simulink subsystem "HI_SPI"  (R2019b)
settings: Solver=VariableStepAuto  StartTime=0.0  StopTime=10.0  RelTol=1e-3
libraries: hdlsllib x1, c280xlib x1
settings Model: Creator=Nick  LastModifiedBy=Nick

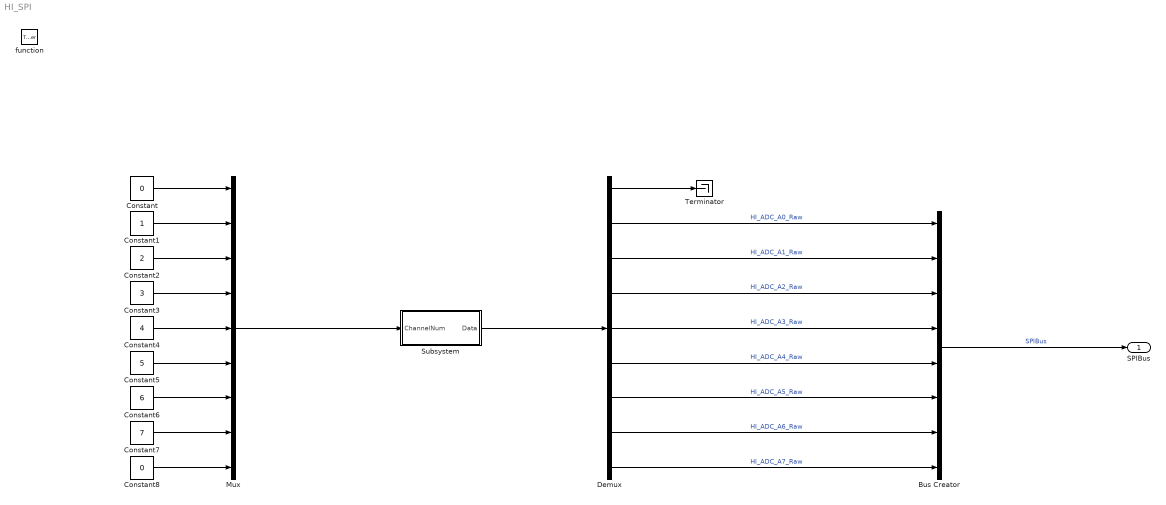
== system HI_SPI ==
  function : TriggerPort  TriggerType=function-call  VariantControl=Variant
  Bus Creator : BusCreator  Inputs=8
  Constant : Constant  Value=0
  Constant1 : Constant
  Constant2 : Constant  Value=2
  Constant3 : Constant  Value=3
  Constant4 : Constant  Value=4
  Constant5 : Constant  Value=5
  Constant6 : Constant  Value=6
  Constant7 : Constant  Value=7
  Constant8 : Constant  Value=0
  Demux : Demux  Outputs=9
  Mux : Mux  Inputs=9
  Subsystem : Subsystem
  Terminator : Terminator
  SPIBus : Outport
  wires:
  Demux/9 -> Bus Creator/8  "HI_ADC_A7_Raw"
  Demux/8 -> Bus Creator/7  "HI_ADC_A6_Raw"
  Demux/7 -> Bus Creator/6  "HI_ADC_A5_Raw"
  Demux/6 -> Bus Creator/5  "HI_ADC_A4_Raw"
  Demux/5 -> Bus Creator/4  "HI_ADC_A3_Raw"
  Demux/4 -> Bus Creator/3  "HI_ADC_A2_Raw"
  Demux/3 -> Bus Creator/2  "HI_ADC_A1_Raw"
  Demux/2 -> Bus Creator/1  "HI_ADC_A0_Raw"
  Demux/1 -> Terminator/1
  Subsystem/1(Data) -> Demux/1
  Mux/1 -> Subsystem/1(ChannelNum)
  Constant8/1 -> Mux/9
  Constant7/1 -> Mux/8
  Constant6/1 -> Mux/7
  Constant5/1 -> Mux/6
  Constant4/1 -> Mux/5
  Constant/1 -> Mux/1
  Constant1/1 -> Mux/2
  Constant2/1 -> Mux/3
  Constant3/1 -> Mux/4
  Bus Creator/1 -> SPIBus/1  "SPIBus"

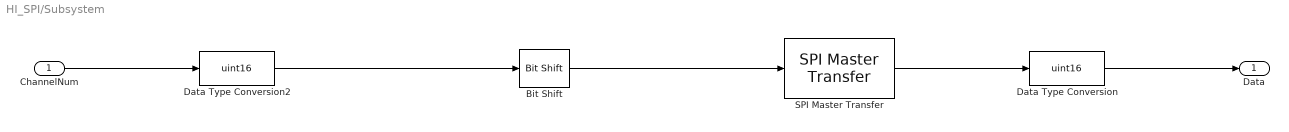
== system HI_SPI/Subsystem ==
  ChannelNum : Inport
  Bit Shift : hdlsllib/Logic and Bit Operations/Bit Shift  mode=Shift Left Logical  N=11
      settings: SourceProductName=Simulink
  Data Type Conversion : DataTypeConversion  OutDataTypeStr=uint16
  Data Type Conversion2 : DataTypeConversion  OutDataTypeStr=uint16
  SPI Master Transfer : c280xlib/SPI Master Transfer  SPISelect=SPI_B  ClockPolarity=Falling_edge  ClockPhase=No_delay  SPIModule=uint32(0)  Mode=Master  BusSpeed=uint32(1000000)  FirstBitToTransfer=Most significant bit (MSB)  ClockMode=0  BlockFunction=Transfer  EnableRegisterAddress=on  RegisterAddress=0  OutputDataType=int8  OutputDataLength=1  DataBits=16  UseCustomSSPin=Explicit GPIO calls  ActiveLowSSPin=Active low  Pin=66
      settings: SourceProductName=Embedded Coder Support Package for Texas Instruments C2000 Processors  SourceProductBaseCode=TIC2000
  Data : Outport
  wires:
  ChannelNum/1 -> Data Type Conversion2/1
  Data Type Conversion/1 -> Data/1
  SPI Master Transfer/1 -> Data Type Conversion/1
  Data Type Conversion2/1 -> Bit Shift/1
  Bit Shift/1 -> SPI Master Transfer/1
